simulink model "exm070101"  (R2018a)
settings: Solver=VariableStepAuto  StartTime=0.0  StopTime=5  MaxStep=0.01  RelTol=1e-3
settings Model: Creator=zyzhang  LastModifiedBy=zyzhang
settings DataIOCC: Refine=10

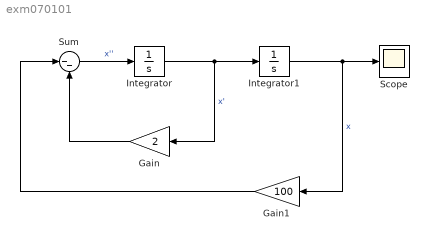
== system exm070101 ==
  Gain : Gain  Gain=2
  Gain1 : Gain  Gain=100
  Integrator : Integrator
  Integrator1 : Integrator  InitialCondition=0.05
  Scope : Scope
  Sum : Sum  Inputs=|--
  wires:
  Sum/1 -> Integrator/1  "x''"
  Integrator/1 -> Gain/1, Integrator1/1  "x'"
  Integrator1/1 -> Gain1/1, Scope/1  "x"
  Gain/1 -> Sum/2
  Gain1/1 -> Sum/1
